simulink model "Practica4"  (R2019b)
settings: Solver=VariableStepAuto  StartTime=0.0  StopTime=10  RelTol=1e-3
undefined symbols (not defined in the file or in its folder): X, Y, Z
libraries: nesl_utility x5, sm_lib x5
settings Model: Creator=Usuario  LastModifiedBy=Usuario

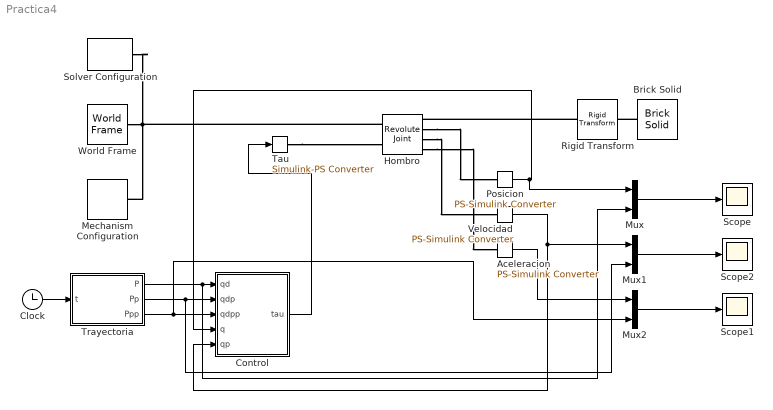
== system Practica4 ==
  Aceleracion : nesl_utility/PS-Simulink Converter  PhysicalDomain=network_engine_domain  SubClassName=ps_output  LeftPortType=input  RightPortType=output  PseudoPeriodic=off  Frequencies=[]  Unit=rad/s^2  AffineConversion=off
  Brick Solid : sm_lib/Body Elements/Brick Solid  GraphicAmbientColor=[0.15 0.15 0.15 1.0]  BasedOnType=Density  BrickDimensions=[0.1 1 0.1]  BrickDimensionUnits=m  CenterOfMass=[0 0 0]  CenterOfMassUnits=m  GraphicDiffuseColor=[0.2 0.2 1.0]  Density=1000  DensityUnits=kg/m^3  DoExposeReferenceFrame=on  GraphicEmissiveColor=[0.0 0.0 0.0 1.0]  ExportEntireGeometry=off  SerializedFrames=<Frames/>  MarkerShape=Sphere  MarkerSize=10  GraphicType=FromGeometry  InertiaType=Custom  Mass=1.1  MassUnits=kg  MomentsOfInertia=[1 1 1]  MomentsOfInertiaUnits=kg*m^2  GraphicOpacity=1.0  ProductsOfInertia=[0 0 0]  ProductsOfInertiaUnits=kg*m^2  GraphicShininess=75  GraphicSpecularColor=[0.5 0.5 0.5 1.0]  GraphicVisPropType=SimpleVisualProperties
  Clock : Clock
  Control : MATLAB Function  TreatAsAtomicUnit=on
  Hombro : sm_lib/Joints/Revolute Joint  JointMode=Normal  SenseConstraintForce=off  SenseConstraintForceX=off  SenseConstraintForceY=off  SenseConstraintForceZ=off  SenseConstraintTorque=off  SenseConstraintTorqueX=off  SenseConstraintTorqueY=off  SenseConstraintTorqueZ=off  SenseTotalForce=off  SenseTotalForceX=off  SenseTotalForceY=off  SenseTotalForceZ=off  SenseTotalTorque=off  SenseTotalTorqueX=off  SenseTotalTorqueY=off  SenseTotalTorqueZ=off  CompositeWrenchDir=FollowerOnBase  CompositeWrenchFrame=BaseFrame  EquilibriumPosition=0  EquilibriumPositionUnits=deg  SpringStiffness=0  SpringStiffnessUnits=N*m/deg  DampingCoefficient=0.003  DampingCoefficientUnits=N*m/(rad/s)  TorqueActuationMode=InputTorque  MotionActuationMode=ComputedMotion  SensePosition=on  SenseVelocity=on  SenseAcceleration=on  SenseTorqueForce=off  SenseLowerLimitTorqueForce=off  SenseUpperLimitTorqueForce=off  LowerLimitSpecify=off  LowerLimitBound=-90  LowerLimitBoundUnits=deg  LowerLimitStiffness=1e4  LowerLimitStiffnessUnits=N*m/deg  LowerLimitDamping=10  LowerLimitDampingUnits=N*m/(deg/s)  LowerLimitTransitionRegionWidth=0.1  LowerLimitTransitionRegionWidthUnits=deg  UpperLimitSpecify=off  UpperLimitBound=90  UpperLimitBoundUnits=deg  UpperLimitStiffness=1e4  UpperLimitStiffnessUnits=N*m/deg  UpperLimitDamping=10  UpperLimitDampingUnits=N*m/(deg/s)  UpperLimitTransitionRegionWidth=0.1  UpperLimitTransitionRegionWidthUnits=deg  PositionTargetSpecify=off  PositionTargetPriority=High  PositionTargetValue=0  PositionTargetValueUnits=deg  VelocityTargetSpecify=off  VelocityTargetPriority=High  VelocityTargetValue=0  VelocityTargetValueUnits=deg/s
  Mechanism Configuration : sm_lib/Utilities/Mechanism Configuration  UniformGravity=Constant  GravityVector=[0 -9.80665 0]  GravityUnits=m/s^2  LinearizationDelta=0.001
  Mux : Mux  Inputs=2
  Mux1 : Mux  Inputs=2
  Mux2 : Mux  Inputs=2
  Posicion : nesl_utility/PS-Simulink Converter  PhysicalDomain=network_engine_domain  SubClassName=ps_output  LeftPortType=input  RightPortType=output  PseudoPeriodic=off  Frequencies=[]  Unit=rad  AffineConversion=off
  Rigid Transform : sm_lib/Frames and Transforms/Rigid Transform  TranslationMethod=Cartesian  TranslationStandardOffset=0  TranslationLengthUnit=m  TranslationStandardAxis=+Z  TranslationCartesianOffset=[0 -0.5 0]  TranslationROffset=0  TranslationROffsetUnits=m  TranslationZOffset=0  TranslationZOffsetUnits=m  TranslationThetaOffset=0  TranslationThetaOffsetUnits=deg  RotationMethod=None  RotationAngleUnits=deg  RotationStandardAxis=+Z  RotationAngle=0.0  RotationArbitraryAxis=[0 0 1]  FollAlignAxisA=+X  BaseAlignAxisA=+Y  FollAlignAxisB=+Y  BaseAlignAxisB=+Z  RotationSequenceAxes=FollowerAxes  RotationSequence=XYX  RotationSequenceAngles=[0 0 0]  RotationSequenceAnglesUnits=deg  RotationMatrix=[1 0 0; 0 1 0; 0 0 1]
  Scope : Scope
  Scope1 : Scope
  Scope2 : Scope
  Solver Configuration : nesl_utility/Solver Configuration  PhysicalDomain=network_engine_domain  SubClassName=solver  LeftPortType=input  RightPortType=generic  Tones=[]  Harmonics=[]  SimulateNoise=off  Profile=off  UseLocalSampling=off  EnableSwitchedLinearOptims=on  FrequencyDomain=off  UseCCode=off  RelTol=0.001  AbsTol=1e-06  MinStep=1e-09  ToWorkspace=off  RevertToSquareIcSolve=off  NumHomotopyIterations=100  PhasorMode=off  PhasorModeNumHarmonics=1  DoDC=off  ResidualTolerance=1e-09  UseLocalSolver=off  LocalSolverChoice=NE_BACKWARD_EULER_ADVANCER  LocalSolverSampleTime=0.001  DoFixedCost=off  MaxNonlinIter=3  MaxModeIter=2  LinearAlgebra=auto  EquationFormulation=NE_TIME_EF  DelaysMemoryBudget=1024  AutomaticFiltering=on  FilteringTimeConstant=0.001  PartitionStorageMethod=AS_NEEDED  PartitionMemoryBudget=1024  PartitionMethod=ROBUST
  Tau : nesl_utility/Simulink-PS Converter  PhysicalDomain=network_engine_domain  SubClassName=ps_input  LeftPortType=input  RightPortType=output  PseudoPeriodic=off  Frequencies=[]  NoiseDistribution=none  NoiseParameters=[]  Unit=1  AffineConversion=off  FilteringAndDerivatives=provide  SimscapeFilterOrder=1  InputFilterTimeConstant=0.001  UdotUserProvided=0
  "Trayectoria " : MATLAB Function  TreatAsAtomicUnit=on
  Velocidad : nesl_utility/PS-Simulink Converter  PhysicalDomain=network_engine_domain  SubClassName=ps_output  LeftPortType=input  RightPortType=output  PseudoPeriodic=off  Frequencies=[]  Unit=rad/s  AffineConversion=off
  World Frame : sm_lib/Frames and Transforms/World Frame
  wires:
  Clock/1 -> "Trayectoria "/1(t)
  Posicion/1 -> Mux/1, Control/4(q)
  Velocidad/1 -> Mux1/1, Control/5(qp)
  "Trayectoria "/1(P) -> Mux/2, Control/1(qd)
  "Trayectoria "/2(Pp) -> Mux1/2, Control/2(qdp)
  "Trayectoria "/3(Ppp) -> Mux2/2, Control/3(qdpp)
  Control/1(tau) -> Tau/1
  Mux/1 -> Scope/1
  Mux1/1 -> Scope2/1
  Mux2/1 -> Scope1/1
  Aceleracion/1 -> Mux2/1
  connections:
  World Frame/RConn1 -- Mechanism Configuration/RConn1 -- Solver Configuration/RConn1 -- Hombro/LConn1
  Rigid Transform/LConn1 -- Hombro/RConn1
  Brick Solid/RConn1 -- Rigid Transform/RConn1
  Hombro/RConn2 -- Posicion/LConn1
  Hombro/RConn3 -- Velocidad/LConn1
  Hombro/RConn4 -- Aceleracion/LConn1
  Tau/RConn1 -- Hombro/LConn2

== matlab function Practica4/Control ==
  data: qd input; tau output; qdp input; qdpp input; q input; qp input
function tau = fcn(qd,qdp,qdpp,q,qp)
%Parametros
m=1;
lc=0.5;
I=1;
g=9.81;
B=0.003;
qh=qd-q;
qhp=qdp-qp;
kp=1;
kd=1;
%Control pd+
tau=kp*qh+kd*qhp+(m*lc^2+I)*qdpp+B*qdpp+m*g*lc*sin(q);
%%Control de par calculado
%%tau=(m*lc^2+I)*(qdpp+kp*qh+kd*qhp)+B*qdpp+m*g*lc*sin(q);

== matlab function Practica4/Trayectoria  ==
  data: t input; P output; Pp output; Ppp output
function [P,Pp,Ppp] = fcn(t)
%%Parametros
teta0=0;
tetaf=pi/2;
teta0p=0;
tetafp=0;
teta0pp=0;
tetafpp=0;
tf=10;
%%Coeficientes
a0=teta0;
a1=teta0p;
a2=teta0pp/2;
a3=(20*tetaf-20*teta0-(8*tetafp+12*teta0p)*tf-(3*teta0pp-tetafpp)*tf^2)/(2*tf^3);
a4=(30*teta0-30*tetaf+(14*tetafp+16*teta0p)*tf+(3*teta0pp-2*tetafpp)*tf^2)/(2*tf^4);
a5=(12*tetaf-12*teta0-(6*tetafp+6*teta0p)*tf-(teta0pp-tetafpp)*tf^2)/(2*tf^5);

%%Polinomio de 5 grado
if t<=tf
P = a0+a1*t+a2*t^2+a3*t^3+a4*t^4+a5*t^5;
Pp = a1+2*a2*t+3*a3*t^2+4*a4*t^3+5*a5*t^4;
Ppp = 2*a2+6*a3*t+12*a4*t^2+20*a5*t^3;
else
    P=tetaf;
    Pp=tetafp;
    Ppp=tetafpp;
end
